simulink model "DetailedModel"  (R2024b)
settings: Solver=ode23t  StartTime=0.0  StopTime=0.2  MaxStep=1e-6  RelTol=1e-4
InitFcn:
  | ModelParameters
undefined symbols (not defined in the file or in its folder): ABR, abr, dc, dc_vs, h_BTU, inv, L, setpoint, Setpoint_Harmonic_L1, time, ts, Ts_RMS
libraries: spsThreePhaseSeriesRLCBranchLib x17, spsGroundLib x14, spsControlledVoltageSourceLib x11, spsThreePhaseVIMeasurementLib x8, spsSeriesRLCBranchLib x7, eePwmGenerator x6, spsCurrentMeasurementLib x4, spsVoltageMeasurementLib x4, spsControlledCurrentSourceLib x3, eePowerMeasurement x3, spsUniversalBridgeLib x2, spsThreePhaseBreakerLib x1
(part 1 of 3)
settings Model: SimulationMode=accelerator  Creator=hw  LastModifiedBy=santh
settings SolverCC: MaxConsecutiveMinStep=10  ShapePreserveControl=EnableAll
settings OptimizationCC: ReuseModelBlockBuffer=off
settings DebuggingCC: UnconnectedInputMsg=warning  UnconnectedOutputMsg=warning  UnconnectedLineMsg=warning
settings ModelReferenceCC: EnableRefExpFcnMdlSchedulingChecks=on
settings RTWCC: GPUComputeCapability=3.5  DLArmComputeVersion=19.05

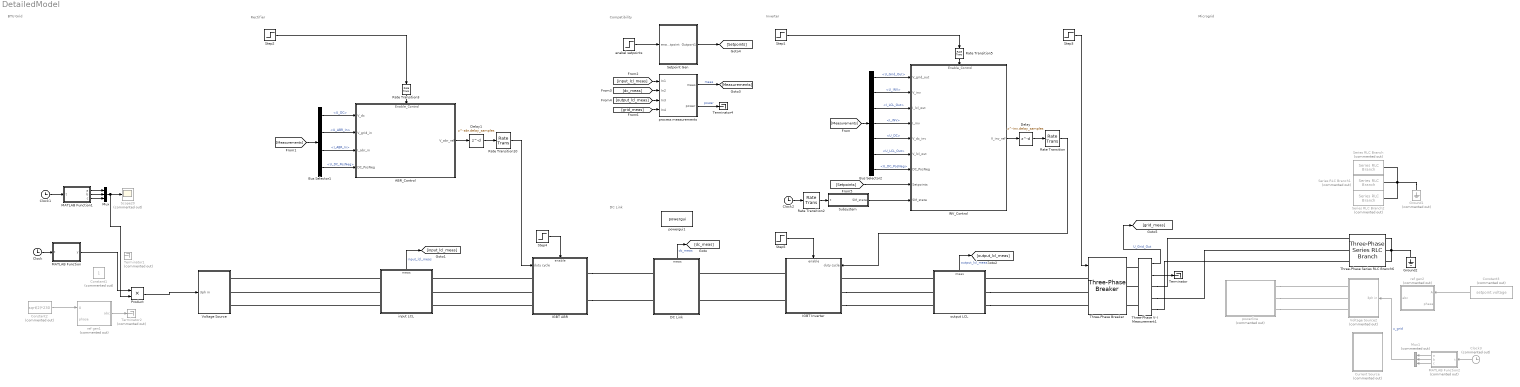
== system DetailedModel ==
  note: Inverter
  note: Rectifier
  note: DC Link
  note: Microgrid
  note: BTU Grid
  note: Compatibility
  " powerline" : Subsystem  Commented=on  Variant=on  VariantControl=Choice
  ABR_Control : Subsystem  Variant=on
      settings: PortSchema="{\"entries\":[{\"content\":{\"sides\":[{\"content\":{\"connectorIds\":[\"In1\",\"In2\",\"In3\",\"In4\"]},\"type\":\"ConnectorPlacement.EquallySpacedRectSide\",\"uuid\":\"9a61e9a7-e233-4fff-bbb7-09c50b9bf7c3\"},{\"content\":{\"connectorIds\":[\"Out1\"],\"side\":\"RIGHT\"},\"type\":\"ConnectorPlacement.EquallySpacedRectSide\",\"uuid\":\"8c6878d7-682c-4532-9753-a6ad9d7eb284\"},{\"content\":{\"connectorIds\":[\"In5\"],\"side\":\"TOP\"},\"type\":\"ConnectorPlacement.EquallySpacedRectSide\",\"uuid\":\"7bdbe081-6677-4104-aee9-21ab386df38d\"}]},\"type\":\"ConnectorPlacement.EquallySpacedConnector\",\"uuid\":\"4e4d951e-f80f-4270-9482-a2bd8c4de465\"}],\"packageUris\":[\"http://schema.mathworks.com/mf0/Connector/R2020b\"],\"version\":\"1.0\"}"
  Bus Selector1 : BusSelector  OutputSignals=U_DC,U_ABR_In,I_ABR_In,U_DC_PosNeg
  Bus Selector2 : BusSelector  OutputSignals=U_Grid_Out,U_INV,I_LCL_Out,I_INV,U_DC,U_LCL_Out,U_DC_PosNeg
  Clock : Clock
  Clock1 : Clock
  Clock2 : Clock
  Clock3 : Clock  Commented=on
  Constant1 : Constant  Commented=on
  Constant2 : Constant  Commented=on  Value=sqrt(2)*230
  Constant3 : Constant  Commented=on  Value=setpoint.voltage
  Current Source : Subsystem  Commented=on  VariantControl=simulate_abr == true;
  DC Link : Subsystem  Variant=on  VariantControl=Choice
      settings: PortSchema="{\"entries\":[{\"content\":{\"sides\":[{\"content\":{\"connectorIds\":[\"LConn1\",\"LConn2\"]},\"type\":\"ConnectorPlacement.EquallySpacedRectSide\",\"uuid\":\"f6ba536e-5264-4926-8f4c-6c75b8afc572\"},{\"content\":{\"connectorIds\":[\"RConn1\",\"RConn2\"],\"side\":\"RIGHT\"},\"type\":\"ConnectorPlacement.EquallySpacedRectSide\",\"uuid\":\"a945ca90-e57b-4883-aff8-0ec279b8e021\"},{\"content\":{\"connectorIds\":[\"Out1\"],\"side\":\"TOP\"},\"type\":\"ConnectorPlacement.EquallySpacedRectSide\",\"uuid\":\"231489ed-e064-4a11-8690-f7178652e5df\"}]},\"type\":\"ConnectorPlacement.EquallySpacedConnector\",\"uuid\":\"69bf4267-a91a-48de-830b-5c3504f7f15c\"}],\"packageUris\":[\"http://schema.mathworks.com/mf0/Connector/R2020b\"],\"version\":\"1.0\"}"
  Delay : Delay  DelayLength=inv.delay_samples
  Delay1 : Delay  DelayLength=abr.delay_samples  SampleTime=h_BTU
  Ground1 : spsGroundLib/Ground  Commented=on  LConnTagsString=a
  Ground2 : spsGroundLib/Ground  LConnTagsString=a
  IGBT ABR : Subsystem  Variant=on  VariantControl=Choice
      settings: PortSchema="{\"entries\":[{\"content\":{\"sides\":[{\"content\":{\"connectorIds\":[\"In1\",\"LConn1\",\"LConn2\",\"LConn3\"]},\"type\":\"ConnectorPlacement.EquallySpacedRectSide\",\"uuid\":\"bdcb7c3b-245c-484b-966a-d1c0a18a3503\"},{\"content\":{\"connectorIds\":[\"RConn1\",\"RConn2\"],\"side\":\"RIGHT\"},\"type\":\"ConnectorPlacement.EquallySpacedRectSide\",\"uuid\":\"68367abd-d947-47d9-a9fd-57ab46e42857\"},{\"content\":{\"connectorIds\":[\"In2\"],\"side\":\"TOP\"},\"type\":\"ConnectorPlacement.EquallySpacedRectSide\",\"uuid\":\"ac48e4a4-8372-427d-a930-cd7797fb7ffc\"}]},\"type\":\"ConnectorPlacement.EquallySpacedConnector\",\"uuid\":\"996b3671-85aa-4bcb-92b7-447b7580701f\"}],\"packageUris\":[\"http://schema.mathworks.com/mf0/Connector/R2020b\"],\"version\":\"1.0\"}"
  IGBT Inverter : Subsystem  Variant=on  VariantControl=Choice
      settings: PortSchema="{\"entries\":[{\"content\":{\"sides\":[{\"content\":{\"connectorIds\":[\"LConn1\",\"LConn2\"]},\"type\":\"ConnectorPlacement.EquallySpacedRectSide\",\"uuid\":\"bdcb7c3b-245c-484b-966a-d1c0a18a3503\"},{\"content\":{\"connectorIds\":[\"In2\",\"RConn1\",\"RConn2\",\"RConn3\"],\"side\":\"RIGHT\"},\"type\":\"ConnectorPlacement.EquallySpacedRectSide\",\"uuid\":\"68367abd-d947-47d9-a9fd-57ab46e42857\"},{\"content\":{\"connectorIds\":[\"In1\"],\"side\":\"TOP\"},\"type\":\"ConnectorPlacement.EquallySpacedRectSide\",\"uuid\":\"ac48e4a4-8372-427d-a930-cd7797fb7ffc\"}]},\"type\":\"ConnectorPlacement.EquallySpacedConnector\",\"uuid\":\"996b3671-85aa-4bcb-92b7-447b7580701f\"}],\"packageUris\":[\"http://schema.mathworks.com/mf0/Connector/R2020b\"],\"version\":\"1.0\"}"
  INV_Control : Subsystem  Variant=on
      settings: PortSchema="{\"entries\":[{\"content\":{\"sides\":[{\"content\":{\"connectorIds\":[\"In1\",\"In2\",\"In3\",\"In4\",\"In5\",\"In6\",\"In7\",\"In8\",\"In9\"]},\"type\":\"ConnectorPlacement.EquallySpacedRectSide\",\"uuid\":\"23e1e123-a779-4f69-b19b-2523a1761b0a\"},{\"content\":{\"connectorIds\":[\"Out1\"],\"side\":\"RIGHT\"},\"type\":\"ConnectorPlacement.EquallySpacedRectSide\",\"uuid\":\"bea06d0c-6610-4352-b580-d1a9b208a554\"},{\"content\":{\"connectorIds\":[\"In10\"],\"side\":\"TOP\"},\"type\":\"ConnectorPlacement.EquallySpacedRectSide\",\"uuid\":\"8bb6373a-e28d-4132-b828-762de06cd811\"}]},\"type\":\"ConnectorPlacement.EquallySpacedConnector\",\"uuid\":\"f1eae18b-7dfa-472c-b275-c02a5c1bef51\"}],\"packageUris\":[\"http://schema.mathworks.com/mf0/Connector/R2020b\"],\"version\":\"1.0\"}"
  MATLAB Function : MATLAB Function  TreatAsAtomicUnit=on
  MATLAB Function1 : MATLAB Function  TreatAsAtomicUnit=on
  MATLAB Function2 : MATLAB Function  Commented=on  TreatAsAtomicUnit=on
  Mux : Mux  Inputs=3
  Mux1 : Mux  Commented=on  Inputs=3
  Product : Product
  Rate Transition : RateTransition
  Rate Transition10 : RateTransition
  Rate Transition2 : RateTransition
  Rate Transition3 : RateTransition  OutPortSampleTime=h_BTU
  Rate Transition5 : RateTransition  OutPortSampleTime=h_BTU
  Scope20 : Scope  Commented=on
  Series RLC Branch : spsSeriesRLCBranchLib/Series RLC Branch  Commented=on  LConnTagsString=__new0  RConnTagsString=__new0  BranchType=R  Resistance=50  Inductance=1e-3  SetiL0=off  InitialCurrent=0  Capacitance=1e-6  Setx0=off  InitialVoltage=0  Measurements=None
  Series RLC Branch1 : spsSeriesRLCBranchLib/Series RLC Branch  Commented=on  LConnTagsString=__new0  RConnTagsString=__new0  BranchType=R  Resistance=40  Inductance=1e-3  SetiL0=off  InitialCurrent=0  Capacitance=1e-6  Setx0=off  InitialVoltage=0  Measurements=None
  Series RLC Branch2 : spsSeriesRLCBranchLib/Series RLC Branch  Commented=on  LConnTagsString=__new0  RConnTagsString=__new0  BranchType=R  Resistance=50  Inductance=1e-3  SetiL0=off  InitialCurrent=0  Capacitance=1e-6  Setx0=off  InitialVoltage=0  Measurements=None
  Setpoint Gen : Subsystem
  Step1 : Step  Time=time.enable_inv_ctrl  SampleTime=0
  Step2 : Step  Time=time.enable_abr_ctrl  SampleTime=0
  Step3 : Step  Time=time.ongrid  SampleTime=0
  Step4 : Step  Time=time.enable_abr  SampleTime=0
  Step5 : Step  Time=time.enable_inv  SampleTime=0
  Subsystem : Subsystem
  Terminator : Terminator
  Terminator1 : Terminator  Commented=on
  Terminator2 : Terminator  Commented=on
  Terminator4 : Terminator
  Three-Phase Series RLC Branch6 : spsThreePhaseSeriesRLCBranchLib/Three-Phase Series RLC Branch  LConnTagsString=A|B|C  RConnTagsString=A|B|C  BranchType=R  Resistance=30  Inductance=350e-6  Capacitance=1e-6  Measurements=None
  Three-Phase V-I Measurement1 : spsThreePhaseVIMeasurementLib/Three-Phase V-I Measurement  VoltageMeasurement=phase-to-ground  SetLabelV=off  LabelV=Vabc  Vpu=off  VpuLL=off  CurrentMeasurement=yes  SetLabelI=off  LabelI=Iabc  Ipu=off  Pbase=100e6  Vbase=500e3  OutputType=Complex  PhasorSimulation=off  PSBequivalent=0
  Three-Phase Breaker : spsThreePhaseBreakerLib/Three-Phase Breaker  InitialState=open  SwitchA=on  SwitchB=on  SwitchC=on  SwitchTimes="[1/60  5/60]"  External=on  BreakerResistance=0.1  SnubberResistance=1e6  SnubberCapacitance=inf  Measurements=None
  Voltage Source : Subsystem  Variant=on  VariantControl=Choice
  Voltage Source2 : Subsystem  Commented=on  VariantControl=simulate_abr == true;
      settings: PortSchema="{\"entries\":[{\"content\":{\"sides\":[{\"content\":{\"connectorIds\":[\"LConn1\",\"LConn2\",\"LConn3\"]},\"type\":\"ConnectorPlacement.EquallySpacedRectSide\",\"uuid\":\"03f06ac6-5cda-41d3-8d94-d4be306d6c6c\"},{\"content\":{\"connectorIds\":[\"In1\"],\"side\":\"RIGHT\"},\"type\":\"ConnectorPlacement.EquallySpacedRectSide\",\"uuid\":\"25d0cb82-e7bd-47db-a03d-611ee4e9a2ac\"},{\"content\":{\"connectorIds\":[],\"side\":\"TOP\"},\"type\":\"ConnectorPlacement.EquallySpacedRectSide\",\"uuid\":\"5bc056cf-5a04-4b34-9ba8-c295df1bce71\"}]},\"type\":\"ConnectorPlacement.EquallySpacedConnector\",\"uuid\":\"225a5fad-493a-40a0-8bfd-b7e904e8dae9\"}],\"packageUris\":[\"http://schema.mathworks.com/mf0/Connector/R2020b\"],\"version\":\"1.0\"}"
  enabel setpoints : Step  Time=time.enable_inv_ctrl  SampleTime=0
  input LCL : Subsystem  Variant=on  VariantControl=Choice
      settings: PortSchema="{\"entries\":[{\"content\":{\"sides\":[{\"content\":{\"connectorIds\":[\"LConn1\",\"LConn2\",\"LConn3\"]},\"type\":\"ConnectorPlacement.EquallySpacedRectSide\",\"uuid\":\"821f425e-e552-4ea9-bdc4-096374f22f7c\"},{\"content\":{\"connectorIds\":[\"RConn1\",\"RConn2\",\"RConn3\"],\"side\":\"RIGHT\"},\"type\":\"ConnectorPlacement.EquallySpacedRectSide\",\"uuid\":\"3ae0e517-8127-4f74-840a-b336b04d9f2b\"},{\"content\":{\"connectorIds\":[\"Out1\"],\"side\":\"TOP\"},\"type\":\"ConnectorPlacement.EquallySpacedRectSide\",\"uuid\":\"969cfcf3-2598-4c06-9b10-5553ede7d6aa\"}]},\"type\":\"ConnectorPlacement.EquallySpacedConnector\",\"uuid\":\"6968de17-154b-4bef-80de-0c55e4fc5823\"}],\"packageUris\":[\"http://schema.mathworks.com/mf0/Connector/R2020b\"],\"version\":\"1.0\"}"
  output LCL : Subsystem
      settings: PortSchema="{\"entries\":[{\"content\":{\"sides\":[{\"content\":{\"connectorIds\":[\"LConn1\",\"LConn2\",\"LConn3\"]},\"type\":\"ConnectorPlacement.EquallySpacedRectSide\",\"uuid\":\"821f425e-e552-4ea9-bdc4-096374f22f7c\"},{\"content\":{\"connectorIds\":[\"RConn1\",\"RConn2\",\"RConn3\"],\"side\":\"RIGHT\"},\"type\":\"ConnectorPlacement.EquallySpacedRectSide\",\"uuid\":\"3ae0e517-8127-4f74-840a-b336b04d9f2b\"},{\"content\":{\"connectorIds\":[\"Out1\"],\"side\":\"TOP\"},\"type\":\"ConnectorPlacement.EquallySpacedRectSide\",\"uuid\":\"969cfcf3-2598-4c06-9b10-5553ede7d6aa\"}]},\"type\":\"ConnectorPlacement.EquallySpacedConnector\",\"uuid\":\"6968de17-154b-4bef-80de-0c55e4fc5823\"}],\"packageUris\":[\"http://schema.mathworks.com/mf0/Connector/R2020b\"],\"version\":\"1.0\"}"
  powergui1 : spspowerguiLib/powergui  Priority=1  SimulationMode=Continuous  SampleTime=h_BTU/100  frequency=60  Iterations=50  frequencyindice=0  Pbase=100e6  ErrMax=1e-4  UnitsV=kV  UnitsW=MW  buscounter=0  FunctionMessages=off  echomessages=off  EnableUseOfTLC=off  CurrentSourceSwitches=off  DisableSnubberDevices=off  DisableRonSwitches=off  DisableVfSwitches=off  DisplayEquations=off  AutomaticDiscreteSolvers=off  SolverType=Tustin/Backward Euler (TBE)  Interpol=off  ExternalGateDelay=off  methode=off  Ts=100  x0status=blocks  SPID=on  SwTol=0  HookPort=off  NonlinearTolerance=1e-4  nMaxIteration=100  ContinueOnMaxIteration=off  RestoreLinks=warning  ResistiveCurrentMeasurement=off  Frange=[0:2:500]  Ylog=off  Xlog=on  ShowGrid=off  save=off  variable=ZData  structure=0  ZoomFFT=off  StartTime=0.0  cycles=1  DisplayStyle=1  fundamental=60  FreqAxis=off  MaxFrequency=1000  frequencyindicesteady=1  RmsSteady=1  display=off
  process measurements : Subsystem
  ref gen1 : Subsystem  Commented=on
  ref gen2 : Subsystem  Commented=on
  wires:
  Delay/1 -> Rate Transition/1
  Step1/1 -> Rate Transition5/1
  Clock1/1 -> MATLAB Function1/1(t)
  Delay1/1 -> Rate Transition10/1
  MATLAB Function1/3(c) -> Mux/3
  Mux/1 -> Product/2, Scope20/1
  ABR_Control/1(V_abr_ref) -> Delay1/1
  MATLAB Function1/2(b) -> Mux/2
  Constant2/1 -> ref gen1/1(A)
  MATLAB Function1/1(a) -> Mux/1
  Clock/1 -> MATLAB Function/1(t)
  INV_Control/1(V_inv_ref) -> Delay/1
  Step2/1 -> Rate Transition3/1
  Rate Transition5/1 -> INV_Control/10(Enable_Control)
  Rate Transition3/1 -> ABR_Control/5(Enable_Control)
  output LCL/1(meas) -> [output_lcl_meas]  "output_lcl_meas"
  [input_lcl_meas] -> process measurements/1(In1)
  [dc_meas] -> process measurements/2(In2)
  [output_lcl_meas] -> process measurements/3(In3)
  DC Link/1(meas) -> [dc_meas]  "dc_meas"
  Bus Selector2/7 -> INV_Control/7(DC_PosNeg)  "<U_DC_PosNeg>"
  Bus Selector2/1 -> INV_Control/1(V_grid_out)  "<U_Grid_Out>"
  Subsystem/1(SM_state) -> INV_Control/9(SM_state)
  Bus Selector1/1 -> ABR_Control/1(V_dc)  "<U_DC>"
  Bus Selector2/3 -> INV_Control/3(I_lcl_out)  "<I_LCL_Out>"
  Bus Selector2/5 -> INV_Control/5(V_dc_inv)  "<U_DC>"
  Bus Selector1/3 -> ABR_Control/3(I_abr_in)  "<I_ABR_In>"
  Bus Selector2/2 -> INV_Control/2(V_inv)  "<U_INV>"
  Bus Selector1/4 -> ABR_Control/4(DC_PosNeg)  "<U_DC_PosNeg>"
  Bus Selector2/4 -> INV_Control/4(I_inv)  "<I_INV>"
  Bus Selector2/6 -> INV_Control/6(V_lcl_out)  "<U_LCL_Out>"
  [Measurements] -> Bus Selector2/1
  Bus Selector1/2 -> ABR_Control/2(V_grid_in)  "<U_ABR_In>"
  process measurements/1(meas) -> [Measurements]  "meas"
  [Setpoints] -> INV_Control/8(Setpoints)
  [Measurements] -> Bus Selector1/1
  Step3/1 -> Three-Phase Breaker/1
  Setpoint Gen/1(Outport1) -> [Setpoints]
  Three-Phase V-I Measurement1/1 -> [grid_meas]  "U_Grid_Out"
  Three-Phase V-I Measurement1/2 -> Terminator/1
  [grid_meas] -> process measurements/4(In4)
  MATLAB Function/1(y) -> Product/1
  ref gen1/1(abc) -> Terminator2/1
  enabel setpoints/1 -> Setpoint Gen/1(enable_setpoint)
  input LCL/1(meas) -> [input_lcl_meas]  "input_lcl_meas"
  Rate Transition10/1 -> IGBT ABR/1(duty cycle)
  Step4/1 -> IGBT ABR/2(enable)
  Rate Transition2/1 -> Subsystem/1(t)
  Clock2/1 -> Rate Transition2/1
  Constant3/1 -> ref gen2/1(A)
  Mux1/1 -> Voltage Source2/1(3ph in)  "u_grid"
  process measurements/2(power) -> Terminator4/1  "power"
  Step5/1 -> IGBT Inverter/1(enable)
  Rate Transition/1 -> IGBT Inverter/2(duty cycle)
  MATLAB Function2/3(c) -> Mux1/3
  MATLAB Function2/2(b) -> Mux1/2
  MATLAB Function2/1(a) -> Mux1/1
  Clock3/1 -> MATLAB Function2/1(t)
  Product/1 -> Voltage Source/1(3ph in)
  connections:
  Three-Phase Series RLC Branch6/RConn1 -- Ground2/LConn1 -- Three-Phase Series RLC Branch6/RConn2 -- Three-Phase Series RLC Branch6/RConn3
  input LCL/LConn1 -- Voltage Source/RConn1
  input LCL/LConn2 -- Voltage Source/RConn2
  input LCL/LConn3 -- Voltage Source/RConn3
  IGBT ABR/LConn1 -- input LCL/RConn1
  IGBT ABR/LConn2 -- input LCL/RConn2
  IGBT ABR/LConn3 -- input LCL/RConn3
  IGBT ABR/RConn1 -- DC Link/LConn1
  IGBT ABR/RConn2 -- DC Link/LConn2
  Three-Phase V-I Measurement1/LConn1 -- Three-Phase Breaker/RConn1
  Three-Phase V-I Measurement1/LConn2 -- Three-Phase Breaker/RConn2
  Three-Phase V-I Measurement1/LConn3 -- Three-Phase Breaker/RConn3
  Three-Phase V-I Measurement1/RConn1 -- Three-Phase Series RLC Branch6/LConn1
  Three-Phase V-I Measurement1/RConn2 -- Three-Phase Series RLC Branch6/LConn2
  Three-Phase V-I Measurement1/RConn3 -- Three-Phase Series RLC Branch6/LConn3
  " powerline"/RConn1 -- Voltage Source2/LConn1
  " powerline"/RConn2 -- Voltage Source2/LConn2
  IGBT Inverter/LConn1 -- DC Link/RConn1
  IGBT Inverter/LConn2 -- DC Link/RConn2
  " powerline"/RConn3 -- Voltage Source2/LConn3
  Ground1/LConn1 -- Series RLC Branch/RConn1 -- Series RLC Branch1/RConn1 -- Series RLC Branch2/RConn1
  output LCL/LConn1 -- IGBT Inverter/RConn1
  IGBT Inverter/RConn2 -- output LCL/LConn2
  IGBT Inverter/RConn3 -- output LCL/LConn3
  Three-Phase Breaker/LConn1 -- output LCL/RConn1
  output LCL/RConn2 -- Three-Phase Breaker/LConn2
  output LCL/RConn3 -- Three-Phase Breaker/LConn3

== system DetailedModel/ powerline ==
  " 0 km" : Subsystem  VariantControl=pimodel == 0
  " 0.5 km" : Subsystem  VariantControl=pimodel == 0.5  mask{L=16e-6, R=20e-3, C=0.56e-6}
      mask prompts: L "Inductance (L)"; R "Resistance (R)"; C "Shunt Capacitys (C)"
  " 10 km" : Subsystem  VariantControl=pimodel == 10  mask{L=350e-6, R=354e-3, C=12e-6}
      mask prompts: L "Inductance (L)"; R "Resistance (R)"; C "Shunt Capacitys (C)"
  " 15 km" : Subsystem  VariantControl=pimodel == 15  mask{L=550e-6, R=538e-3, C=18e-6}
      mask prompts: L "Inductance (L)"; R "Resistance (R)"; C "Shunt Capacitys (C)"
  A1 : PMIOPort  Side=Left
  B1 : PMIOPort  Port=2  Side=Left
  C1 : PMIOPort  Port=3  Side=Left
  A2 : PMIOPort  Port=4  Side=Right
  B2 : PMIOPort  Port=5  Side=Right
  C2 : PMIOPort  Port=6  Side=Right

== system DetailedModel/ABR_Control ==
  note: 1) Add Subsystem or Model blocks as valid variant choices.
      | 2) You cannot connect blocks at this level. At simulation, connectivity is automatically
      | determined, based on the active variant and port name matching.
  V_dc : Inport
  V_grid_in : Inport  Port=2
  I_abr_in : Inport  Port=3
  DC_PosNeg : Inport  Port=4
  Enable_Control : Inport  Port=5
  PR_no_feedback : Subsystem  VariantControl=simulate_abr==true && ABR_Mode == 3  ReferencedSubsystem=PR_no_feedback
  deactive : Subsystem  VariantControl=simulate_abr == false
  V_abr_ref : Outport

== system DetailedModel/Current Source ==
  Constant3 : Constant  Value=setpoint.voltage
  Controlled Current Source1 : spsControlledCurrentSourceLib/Controlled Current Source  Initialize=on  Source_Type=AC  Amplitude=0  Phase=0  Frequency=0  Measurements=None
  Controlled Current Source2 : spsControlledCurrentSourceLib/Controlled Current Source  Initialize=on  Source_Type=AC  Amplitude=0  Phase=0  Frequency=0  Measurements=None
  Controlled Current Source3 : spsControlledCurrentSourceLib/Controlled Current Source  Initialize=on  Source_Type=AC  Amplitude=0  Phase=0  Frequency=0  Measurements=None
  Demux : Demux  Outputs=3
  Divide : Product  Inputs=*/
  Gain : Gain  Gain=setpoint.current
  Ground : spsGroundLib/Ground  LConnTagsString=a
  Terminator : Terminator
  Three-Phase V-I Measurement : spsThreePhaseVIMeasurementLib/Three-Phase V-I Measurement  VoltageMeasurement=phase-to-ground  SetLabelV=off  LabelV=Vabc  Vpu=off  VpuLL=off  CurrentMeasurement=yes  SetLabelI=off  LabelI=Iabc  Ipu=off  Pbase=100e6  Vbase=500e3  OutputType=Complex  PhasorSimulation=off  PSBequivalent=0
  a : PMIOPort  Side=Left
  b : PMIOPort  Port=2  Side=Left
  c : PMIOPort  Port=3  Side=Left
  wires:
  Gain/1 -> Demux/1
  Demux/3 -> Controlled Current Source3/1
  Demux/2 -> Controlled Current Source2/1
  Demux/1 -> Controlled Current Source1/1
  Three-Phase V-I Measurement/2 -> Terminator/1
  Three-Phase V-I Measurement/1 -> Divide/1
  Constant3/1 -> Divide/2
  Divide/1 -> Gain/1
  connections:
  Ground/LConn1 -- Controlled Current Source1/LConn1 -- Controlled Current Source2/LConn1 -- Controlled Current Source3/LConn1
  Controlled Current Source3/RConn1 -- Three-Phase V-I Measurement/LConn3
  Controlled Current Source2/RConn1 -- Three-Phase V-I Measurement/LConn2
  Controlled Current Source1/RConn1 -- Three-Phase V-I Measurement/LConn1
  a/RConn1 -- Three-Phase V-I Measurement/RConn1
  b/RConn1 -- Three-Phase V-I Measurement/RConn2
  c/RConn1 -- Three-Phase V-I Measurement/RConn3

== system DetailedModel/DC Link ==
  full model : Subsystem  VariantControl=simulate_abr == true;
      settings: PortSchema="{\"entries\":[{\"content\":{\"sides\":[{\"content\":{\"connectorIds\":[\"LConn1\",\"LConn2\"]},\"type\":\"ConnectorPlacement.EquallySpacedRectSide\",\"uuid\":\"f6ba536e-5264-4926-8f4c-6c75b8afc572\"},{\"content\":{\"connectorIds\":[\"RConn1\",\"RConn2\"],\"side\":\"RIGHT\"},\"type\":\"ConnectorPlacement.EquallySpacedRectSide\",\"uuid\":\"a945ca90-e57b-4883-aff8-0ec279b8e021\"},{\"content\":{\"connectorIds\":[\"Out1\"],\"side\":\"TOP\"},\"type\":\"ConnectorPlacement.EquallySpacedRectSide\",\"uuid\":\"231489ed-e064-4a11-8690-f7178652e5df\"}]},\"type\":\"ConnectorPlacement.EquallySpacedConnector\",\"uuid\":\"69bf4267-a91a-48de-830b-5c3504f7f15c\"}],\"packageUris\":[\"http://schema.mathworks.com/mf0/Connector/R2020b\"],\"version\":\"1.0\"}"
  vsource : Subsystem  VariantControl=simulate_abr == false;
      settings: PortSchema="{\"entries\":[{\"content\":{\"sides\":[{\"content\":{\"connectorIds\":[\"LConn1\",\"LConn2\"]},\"type\":\"ConnectorPlacement.EquallySpacedRectSide\",\"uuid\":\"f6ba536e-5264-4926-8f4c-6c75b8afc572\"},{\"content\":{\"connectorIds\":[\"RConn1\",\"RConn2\"],\"side\":\"RIGHT\"},\"type\":\"ConnectorPlacement.EquallySpacedRectSide\",\"uuid\":\"a945ca90-e57b-4883-aff8-0ec279b8e021\"},{\"content\":{\"connectorIds\":[\"Out1\"],\"side\":\"TOP\"},\"type\":\"ConnectorPlacement.EquallySpacedRectSide\",\"uuid\":\"231489ed-e064-4a11-8690-f7178652e5df\"}]},\"type\":\"ConnectorPlacement.EquallySpacedConnector\",\"uuid\":\"69bf4267-a91a-48de-830b-5c3504f7f15c\"}],\"packageUris\":[\"http://schema.mathworks.com/mf0/Connector/R2020b\"],\"version\":\"1.0\"}"
  plus1 : PMIOPort  Side=Left
  minus1 : PMIOPort  Port=2  Side=Left
  plus2 : PMIOPort  Port=3  Side=Right
  minus2 : PMIOPort  Port=4  Side=Right
  meas : Outport

== system DetailedModel/IGBT ABR ==
  duty cycle : Inport
  enable : Inport  Port=2
  IGBT ABR : Subsystem  VariantControl=simulate_abr == true;
      settings: PortSchema="{\"entries\":[{\"content\":{\"sides\":[{\"content\":{\"connectorIds\":[\"In1\",\"LConn1\",\"LConn2\",\"LConn3\"]},\"type\":\"ConnectorPlacement.EquallySpacedRectSide\",\"uuid\":\"bdcb7c3b-245c-484b-966a-d1c0a18a3503\"},{\"content\":{\"connectorIds\":[\"RConn1\",\"RConn2\"],\"side\":\"RIGHT\"},\"type\":\"ConnectorPlacement.EquallySpacedRectSide\",\"uuid\":\"68367abd-d947-47d9-a9fd-57ab46e42857\"},{\"content\":{\"connectorIds\":[\"In2\"],\"side\":\"TOP\"},\"type\":\"ConnectorPlacement.EquallySpacedRectSide\",\"uuid\":\"ac48e4a4-8372-427d-a930-cd7797fb7ffc\"}]},\"type\":\"ConnectorPlacement.EquallySpacedConnector\",\"uuid\":\"996b3671-85aa-4bcb-92b7-447b7580701f\"}],\"packageUris\":[\"http://schema.mathworks.com/mf0/Connector/R2020b\"],\"version\":\"1.0\"}"
  deactivate : Subsystem  VariantControl=simulate_abr == false;
      settings: PortSchema="{\"entries\":[{\"content\":{\"sides\":[{\"content\":{\"connectorIds\":[\"In1\",\"LConn1\",\"LConn2\",\"LConn3\"]},\"type\":\"ConnectorPlacement.EquallySpacedRectSide\",\"uuid\":\"bdcb7c3b-245c-484b-966a-d1c0a18a3503\"},{\"content\":{\"connectorIds\":[\"RConn1\",\"RConn2\"],\"side\":\"RIGHT\"},\"type\":\"ConnectorPlacement.EquallySpacedRectSide\",\"uuid\":\"68367abd-d947-47d9-a9fd-57ab46e42857\"},{\"content\":{\"connectorIds\":[\"In2\"],\"side\":\"TOP\"},\"type\":\"ConnectorPlacement.EquallySpacedRectSide\",\"uuid\":\"ac48e4a4-8372-427d-a930-cd7797fb7ffc\"}]},\"type\":\"ConnectorPlacement.EquallySpacedConnector\",\"uuid\":\"996b3671-85aa-4bcb-92b7-447b7580701f\"}],\"packageUris\":[\"http://schema.mathworks.com/mf0/Connector/R2020b\"],\"version\":\"1.0\"}"
  A : PMIOPort  Side=Left
  B : PMIOPort  Port=2  Side=Left
  C : PMIOPort  Port=3  Side=Left
  DC plus : PMIOPort  Port=4  Side=Right
  DC minus : PMIOPort  Port=5  Side=Right

== system DetailedModel/IGBT Inverter ==
  enable : Inport
  duty cycle : Inport  Port=2
  IGBT Inverter : Subsystem  VariantControl="inv_sim_mode == \"igbt\""
      settings: PortSchema="{\"entries\":[{\"content\":{\"sides\":[{\"content\":{\"connectorIds\":[\"LConn1\",\"LConn2\"]},\"type\":\"ConnectorPlacement.EquallySpacedRectSide\",\"uuid\":\"bdcb7c3b-245c-484b-966a-d1c0a18a3503\"},{\"content\":{\"connectorIds\":[\"In2\",\"RConn1\",\"RConn2\",\"RConn3\"],\"side\":\"RIGHT\"},\"type\":\"ConnectorPlacement.EquallySpacedRectSide\",\"uuid\":\"68367abd-d947-47d9-a9fd-57ab46e42857\"},{\"content\":{\"connectorIds\":[\"In1\"],\"side\":\"TOP\"},\"type\":\"ConnectorPlacement.EquallySpacedRectSide\",\"uuid\":\"ac48e4a4-8372-427d-a930-cd7797fb7ffc\"}]},\"type\":\"ConnectorPlacement.EquallySpacedConnector\",\"uuid\":\"996b3671-85aa-4bcb-92b7-447b7580701f\"}],\"packageUris\":[\"http://schema.mathworks.com/mf0/Connector/R2020b\"],\"version\":\"1.0\"}"
  average model : Subsystem  VariantControl="inv_sim_mode == \"avg\""
      settings: PortSchema="{\"entries\":[{\"content\":{\"sides\":[{\"content\":{\"connectorIds\":[\"LConn1\",\"LConn2\"]},\"type\":\"ConnectorPlacement.EquallySpacedRectSide\",\"uuid\":\"bdcb7c3b-245c-484b-966a-d1c0a18a3503\"},{\"content\":{\"connectorIds\":[\"In2\",\"RConn1\",\"RConn2\",\"RConn3\"],\"side\":\"RIGHT\"},\"type\":\"ConnectorPlacement.EquallySpacedRectSide\",\"uuid\":\"68367abd-d947-47d9-a9fd-57ab46e42857\"},{\"content\":{\"connectorIds\":[\"In1\"],\"side\":\"TOP\"},\"type\":\"ConnectorPlacement.EquallySpacedRectSide\",\"uuid\":\"ac48e4a4-8372-427d-a930-cd7797fb7ffc\"}]},\"type\":\"ConnectorPlacement.EquallySpacedConnector\",\"uuid\":\"996b3671-85aa-4bcb-92b7-447b7580701f\"}],\"packageUris\":[\"http://schema.mathworks.com/mf0/Connector/R2020b\"],\"version\":\"1.0\"}"
  DC plus : PMIOPort  Side=Left
  DC minus : PMIOPort  Port=2  Side=Left
  A : PMIOPort  Port=3  Side=Right
  B : PMIOPort  Port=4  Side=Right
  C : PMIOPort  Port=5  Side=Right

== system DetailedModel/INV_Control ==
  note: 1) Add Subsystem or Model blocks as valid variant choices.
      | 2) You cannot connect blocks at this level. At simulation, connectivity is automatically
      | determined, based on the active variant and port name matching.
  V_grid_out : Inport
  V_inv : Inport  Port=2
  I_lcl_out : Inport  Port=3
  I_inv : Inport  Port=4
  V_dc_inv : Inport  Port=5
  V_lcl_out : Inport  Port=6
  DC_PosNeg : Inport  Port=7
  Setpoints : Inport  Port=8
  SM_state : Inport  Port=9
  Enable_Control : Inport  Port=10
  BTU_DQ_Current_Control : Subsystem  VariantControl=INV_Mode==10  ReferencedSubsystem=BTU_DQ_Current_Control
      settings: PortSchema="{\"entries\":[{\"content\":{\"sides\":[{\"content\":{\"connectorIds\":[\"In9\",\"In10\",\"In1\",\"In2\",\"In3\",\"In4\",\"In5\",\"In6\",\"In7\",\"In8\"]},\"type\":\"ConnectorPlacement.EquallySpacedRectSide\",\"uuid\":\"6baa388e-7184-42e1-a65e-c042756fabf1\"},{\"content\":{\"connectorIds\":[\"Out1\"],\"side\":\"RIGHT\"},\"type\":\"ConnectorPlacement.EquallySpacedRectSide\",\"uuid\":\"9ce0a75c-01ec-48aa-a778-a1584ec40358\"},{\"content\":{\"side\":\"TOP\"},\"type\":\"ConnectorPlacement.EquallySpacedRectSide\",\"uuid\":\"441b7bcf-f48e-499e-91f5-94fbdb47275e\"}]},\"type\":\"ConnectorPlacement.EquallySpacedConnector\",\"uuid\":\"4bbbbfed-a9b6-439f-a0bf-aea6944f8f31\"}],\"packageUris\":[\"http://schema.mathworks.com/mf0/Connector/R2020b\"],\"version\":\"1.0\"}"
  BTU_DQ_Voltage_Control : Subsystem  VariantControl=INV_Mode==9  ReferencedSubsystem=BTU_DQ_Voltage_Control
  BTU_Droop_DQ_based : Subsystem  VariantControl=INV_Mode==11  ReferencedSubsystem=BTU_Droop_DQ_based
      settings: PortSchema="{\"entries\":[{\"content\":{\"sides\":[{\"content\":{\"connectorIds\":[\"In9\",\"In10\",\"In1\",\"In2\",\"In3\",\"In4\",\"In5\",\"In6\",\"In7\",\"In8\"]},\"type\":\"ConnectorPlacement.EquallySpacedRectSide\",\"uuid\":\"6baa388e-7184-42e1-a65e-c042756fabf1\"},{\"content\":{\"connectorIds\":[\"Out1\"],\"side\":\"RIGHT\"},\"type\":\"ConnectorPlacement.EquallySpacedRectSide\",\"uuid\":\"9ce0a75c-01ec-48aa-a778-a1584ec40358\"},{\"content\":{\"side\":\"TOP\"},\"type\":\"ConnectorPlacement.EquallySpacedRectSide\",\"uuid\":\"441b7bcf-f48e-499e-91f5-94fbdb47275e\"}]},\"type\":\"ConnectorPlacement.EquallySpacedConnector\",\"uuid\":\"4bbbbfed-a9b6-439f-a0bf-aea6944f8f31\"}],\"packageUris\":[\"http://schema.mathworks.com/mf0/Connector/R2020b\"],\"version\":\"1.0\"}"
  BTU_PR_Current_Control : Subsystem  VariantControl=INV_Mode==8  ReferencedSubsystem=BTU_PR_Current_Control
  BTU_PR_Voltage_Control : Subsystem  VariantControl=INV_Mode==7  ReferencedSubsystem=BTU_PR_Voltage_Control
  V_inv_ref : Outport

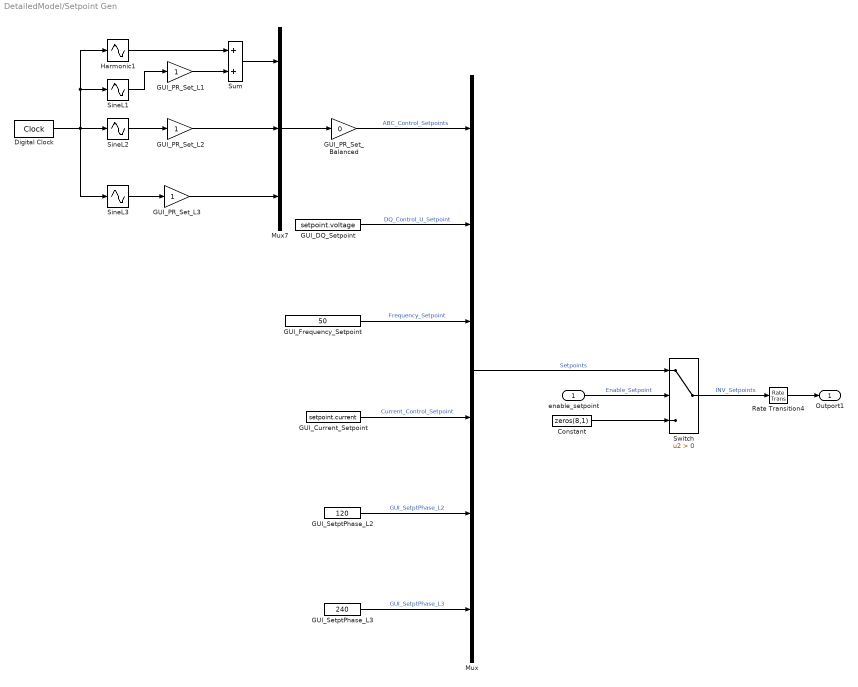
== system DetailedModel/Setpoint Gen ==
  enable_setpoint : Inport
  Constant : Constant  Value=zeros(8,1)  SampleTime=-1
  Digital Clock : DigitalClock  SampleTime=h_BTU
  GUI_Current_Setpoint : Constant  Value=setpoint.current  SampleTime=-1
  GUI_DQ_Setpoint : Constant  Value=setpoint.voltage  SampleTime=-1
  GUI_Frequency_Setpoint : Constant  Value=50  SampleTime=-1
  GUI_PR_Set_Balanced : Gain  Gain=0
  GUI_PR_Set_L1 : Gain
  GUI_PR_Set_L2 : Gain
  GUI_PR_Set_L3 : Gain
  GUI_SetptPhase_L2 : Constant  Value=120  SampleTime=-1
  GUI_SetptPhase_L3 : Constant  Value=240  SampleTime=-1
  Harmonic1 : Sin  TimeSource=Use external signal  Amplitude=Setpoint_Harmonic_L1  Frequency=2*pi*50*7
  Mux : Mux  Inputs=6
  Mux7 : Mux  Inputs=3
  Rate Transition4 : RateTransition  OutPortSampleTime=h_BTU
  SineL1 : Sin  TimeSource=Use external signal  Frequency=2*pi*50
  SineL2 : Sin  TimeSource=Use external signal  Frequency=2*pi*50  Phase=-2*pi/3
  SineL3 : Sin  TimeSource=Use external signal  Frequency=2*pi*50  Phase=-2*pi*2/3
  Sum : Sum
  Switch : Switch  Criteria=u2 > Threshold  SaturateOnIntegerOverflow=off  InputSameDT=off
  Outport1 : Outport
  wires:
  Mux7/1 -> GUI_PR_Set_Balanced/1
  SineL2/1 -> GUI_PR_Set_L2/1
  SineL3/1 -> GUI_PR_Set_L3/1
  SineL1/1 -> GUI_PR_Set_L1/1
  GUI_Current_Setpoint/1 -> Mux/4  "Current_Control_Setpoint"
  GUI_PR_Set_Balanced/1 -> Mux/1  "ABC_Control_Setpoints"
  GUI_PR_Set_L1/1 -> Sum/2
  GUI_PR_Set_L2/1 -> Mux7/2
  GUI_PR_Set_L3/1 -> Mux7/3
  GUI_Frequency_Setpoint/1 -> Mux/3  "Frequency_Setpoint"
  GUI_DQ_Setpoint/1 -> Mux/2  "DQ_Control_U_Setpoint"
  Mux/1 -> Switch/1  "Setpoints"
  Digital Clock/1 -> SineL3/1, Harmonic1/1, SineL1/1, SineL2/1
  Harmonic1/1 -> Sum/1
  Sum/1 -> Mux7/1
  GUI_SetptPhase_L2/1 -> Mux/5  "GUI_SetptPhase_L2"
  GUI_SetptPhase_L3/1 -> Mux/6  "GUI_SetptPhase_L3"
  Constant/1 -> Switch/3
  enable_setpoint/1 -> Switch/2  "Enable_Setpoint"
  Switch/1 -> Rate Transition4/1  "INV_Setpoints"
  Rate Transition4/1 -> Outport1/1

== system DetailedModel/Subsystem ==
  t : Inport
  Constant : Constant  Value=time.ongrid
  Constant1 : Constant  Value=6
  Constant2 : Constant  Value=time.enable_abr
  Constant3 : Constant  Value=5
  Constant4 : Constant  Value=4
  GreaterThanOrEqual : RelationalOperator  OutDataTypeStr=boolean  RndMeth=Simplest  InputSameDT=off
  GreaterThanOrEqual1 : RelationalOperator  OutDataTypeStr=boolean  RndMeth=Simplest  InputSameDT=off
  Switch : Switch  Criteria=u2 > Threshold  SaturateOnIntegerOverflow=off  InputSameDT=off
  Switch1 : Switch  Criteria=u2 > Threshold  SaturateOnIntegerOverflow=off  InputSameDT=off
  SM_state : Outport
  wires:
  Constant/1 -> GreaterThanOrEqual/2
  GreaterThanOrEqual/1 -> Switch/2
  Constant1/1 -> Switch/1
  GreaterThanOrEqual1/1 -> Switch1/2
  Constant3/1 -> Switch1/1
  t/1 -> GreaterThanOrEqual1/1, GreaterThanOrEqual/1
  Constant2/1 -> GreaterThanOrEqual1/2
  Switch1/1 -> Switch/3
  Constant4/1 -> Switch1/3
  Switch/1 -> SM_state/1

== system DetailedModel/Voltage Source ==
  3ph in : Inport
  Voltage Source : Subsystem  VariantControl=simulate_abr == true;
  deactive : Subsystem  VariantControl=simulate_abr == false;
  a : PMIOPort  Side=Right
  b : PMIOPort  Port=2  Side=Right
  c : PMIOPort  Port=3  Side=Right

== system DetailedModel/Voltage Source2 ==
  3ph in : Inport
  Controlled Voltage Source : spsControlledVoltageSourceLib/Controlled Voltage Source  Initialize=on  Source_Type=AC  Amplitude=0  Phase=0  Frequency=0  Measurements=None
  Controlled Voltage Source1 : spsControlledVoltageSourceLib/Controlled Voltage Source  Initialize=on  Source_Type=AC  Amplitude=0  Phase=0  Frequency=0  Measurements=None
  Controlled Voltage Source2 : spsControlledVoltageSourceLib/Controlled Voltage Source  Initialize=on  Source_Type=AC  Amplitude=0  Phase=0  Frequency=0  Measurements=None
  Demux : Demux  Outputs=3
  Ground : spsGroundLib/Ground  LConnTagsString=a
  Three-Phase Series RLC Branch1 : spsThreePhaseSeriesRLCBranchLib/Three-Phase Series RLC Branch  LConnTagsString=A|B|C  RConnTagsString=A|B|C  BranchType=R  Resistance=1e-4  Inductance=L  Capacitance=1e-6  Measurements=None
  a : PMIOPort  Side=Left
  b : PMIOPort  Port=2  Side=Left
  c : PMIOPort  Port=3  Side=Left
  wires:
  3ph in/1 -> Demux/1
  Demux/3 -> Controlled Voltage Source2/1
  Demux/2 -> Controlled Voltage Source1/1
  Demux/1 -> Controlled Voltage Source/1
  connections:
  Three-Phase Series RLC Branch1/LConn3 -- Controlled Voltage Source2/RConn1
  Three-Phase Series RLC Branch1/LConn2 -- Controlled Voltage Source1/RConn1
  Three-Phase Series RLC Branch1/LConn1 -- Controlled Voltage Source/RConn1
  Ground/LConn1 -- Controlled Voltage Source1/LConn1 -- Controlled Voltage Source2/LConn1 -- Controlled Voltage Source/LConn1
  c/RConn1 -- Three-Phase Series RLC Branch1/RConn3
  Three-Phase Series RLC Branch1/RConn2 -- b/RConn1
  Three-Phase Series RLC Branch1/RConn1 -- a/RConn1

== system DetailedModel/input LCL ==
  deactive : Subsystem  VariantControl=simulate_abr == false
      settings: PortSchema="{\"entries\":[{\"content\":{\"sides\":[{\"content\":{\"connectorIds\":[\"LConn1\",\"LConn2\",\"LConn3\"]},\"type\":\"ConnectorPlacement.EquallySpacedRectSide\",\"uuid\":\"821f425e-e552-4ea9-bdc4-096374f22f7c\"},{\"content\":{\"connectorIds\":[\"RConn1\",\"RConn2\",\"RConn3\"],\"side\":\"RIGHT\"},\"type\":\"ConnectorPlacement.EquallySpacedRectSide\",\"uuid\":\"3ae0e517-8127-4f74-840a-b336b04d9f2b\"},{\"content\":{\"connectorIds\":[\"Out1\"],\"side\":\"TOP\"},\"type\":\"ConnectorPlacement.EquallySpacedRectSide\",\"uuid\":\"969cfcf3-2598-4c06-9b10-5553ede7d6aa\"}]},\"type\":\"ConnectorPlacement.EquallySpacedConnector\",\"uuid\":\"6968de17-154b-4bef-80de-0c55e4fc5823\"}],\"packageUris\":[\"http://schema.mathworks.com/mf0/Connector/R2020b\"],\"version\":\"1.0\"}"
  input LCL : Subsystem  VariantControl=simulate_abr == true
      settings: PortSchema="{\"entries\":[{\"content\":{\"sides\":[{\"content\":{\"connectorIds\":[\"LConn1\",\"LConn2\",\"LConn3\"]},\"type\":\"ConnectorPlacement.EquallySpacedRectSide\",\"uuid\":\"821f425e-e552-4ea9-bdc4-096374f22f7c\"},{\"content\":{\"connectorIds\":[\"RConn1\",\"RConn2\",\"RConn3\"],\"side\":\"RIGHT\"},\"type\":\"ConnectorPlacement.EquallySpacedRectSide\",\"uuid\":\"3ae0e517-8127-4f74-840a-b336b04d9f2b\"},{\"content\":{\"connectorIds\":[\"Out1\"],\"side\":\"TOP\"},\"type\":\"ConnectorPlacement.EquallySpacedRectSide\",\"uuid\":\"969cfcf3-2598-4c06-9b10-5553ede7d6aa\"}]},\"type\":\"ConnectorPlacement.EquallySpacedConnector\",\"uuid\":\"6968de17-154b-4bef-80de-0c55e4fc5823\"}],\"packageUris\":[\"http://schema.mathworks.com/mf0/Connector/R2020b\"],\"version\":\"1.0\"}"
  A1 : PMIOPort  Side=Left
  B1 : PMIOPort  Port=2  Side=Left
  C1 : PMIOPort  Port=3  Side=Left
  A2 : PMIOPort  Port=4  Side=Right
  B2 : PMIOPort  Port=5  Side=Right
  C2 : PMIOPort  Port=6  Side=Right
  meas : Outport

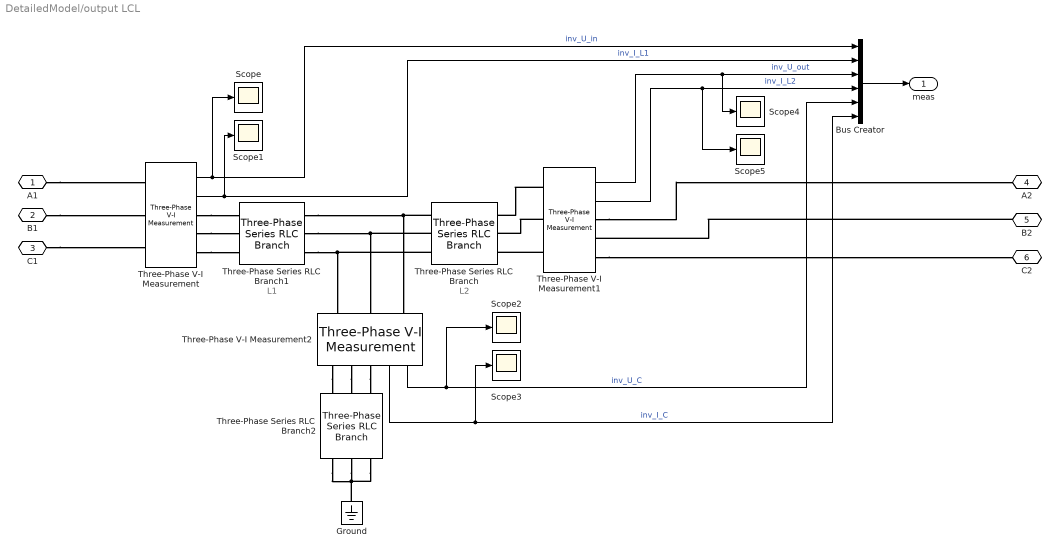
== system DetailedModel/output LCL ==
  note: L2
  note: L1
  Bus Creator : BusCreator  Inputs=6
  Ground : spsGroundLib/Ground  LConnTagsString=a
  Scope{,1..5} (6 alike) : Scope
  Three-Phase Series RLC Branch : spsThreePhaseSeriesRLCBranchLib/Three-Phase Series RLC Branch  LConnTagsString=A|B|C  RConnTagsString=A|B|C  BranchType=RL  Resistance=inv.R2  Inductance=inv.L2  Capacitance=1e-6  Measurements=None
  Three-Phase Series RLC Branch1 : spsThreePhaseSeriesRLCBranchLib/Three-Phase Series RLC Branch  LConnTagsString=A|B|C  RConnTagsString=A|B|C  BranchType=RL  Resistance=inv.R1  Inductance=inv.L1  Capacitance=1e-6  Measurements=None
  Three-Phase Series RLC Branch2 : spsThreePhaseSeriesRLCBranchLib/Three-Phase Series RLC Branch  LConnTagsString=A|B|C  RConnTagsString=A|B|C  BranchType=RC  Resistance=inv.RC  Inductance=13e-6  Capacitance=inv.C  Measurements=None
  Three-Phase V-I Measurement : spsThreePhaseVIMeasurementLib/Three-Phase V-I Measurement  VoltageMeasurement=phase-to-ground  SetLabelV=off  LabelV=Vabc  Vpu=off  VpuLL=off  CurrentMeasurement=yes  SetLabelI=off  LabelI=Iabc  Ipu=off  Pbase=100e6  Vbase=500e3  OutputType=Complex  PhasorSimulation=off  PSBequivalent=0
  Three-Phase V-I Measurement1 : spsThreePhaseVIMeasurementLib/Three-Phase V-I Measurement  VoltageMeasurement=phase-to-ground  SetLabelV=off  LabelV=Vabc  Vpu=off  VpuLL=off  CurrentMeasurement=yes  SetLabelI=off  LabelI=Iabc  Ipu=off  Pbase=100e6  Vbase=500e3  OutputType=Complex  PhasorSimulation=off  PSBequivalent=0
  Three-Phase V-I Measurement2 : spsThreePhaseVIMeasurementLib/Three-Phase V-I Measurement  VoltageMeasurement=phase-to-ground  SetLabelV=off  LabelV=Vabc  Vpu=off  VpuLL=off  CurrentMeasurement=yes  SetLabelI=off  LabelI=Iabc  Ipu=off  Pbase=100e6  Vbase=500e3  OutputType=Complex  PhasorSimulation=off  PSBequivalent=0
  A1 : PMIOPort  Side=Left
  B1 : PMIOPort  Port=2  Side=Left
  C1 : PMIOPort  Port=3  Side=Left
  A2 : PMIOPort  Port=4  Side=Right
  B2 : PMIOPort  Port=5  Side=Right
  C2 : PMIOPort  Port=6  Side=Right
  meas : Outport
  wires:
  Bus Creator/1 -> meas/1
  Three-Phase V-I Measurement1/2 -> Scope5/1, Bus Creator/4  "inv_I_L2"
  Three-Phase V-I Measurement/2 -> Scope1/1, Bus Creator/2  "inv_I_L1"
  Three-Phase V-I Measurement/1 -> Scope/1, Bus Creator/1  "inv_U_in"
  Three-Phase V-I Measurement2/1 -> Scope2/1, Bus Creator/5  "inv_U_C"
  Three-Phase V-I Measurement2/2 -> Scope3/1, Bus Creator/6  "inv_I_C"
  Three-Phase V-I Measurement1/1 -> Scope4/1, Bus Creator/3  "inv_U_out"
  connections:
  Three-Phase V-I Measurement1/RConn3 -- C2/RConn1
  B2/RConn1 -- Three-Phase V-I Measurement1/RConn2
  B1/RConn1 -- Three-Phase V-I Measurement/LConn2
  Three-Phase V-I Measurement2/RConn2 -- Three-Phase Series RLC Branch2/LConn2
  Three-Phase Series RLC Branch/LConn1 -- Three-Phase Series RLC Branch1/RConn1 -- Three-Phase V-I Measurement2/LConn1
  Three-Phase V-I Measurement1/LConn2 -- Three-Phase Series RLC Branch/RConn2
  Three-Phase V-I Measurement2/RConn1 -- Three-Phase Series RLC Branch2/LConn3
  A1/RConn1 -- Three-Phase V-I Measurement/LConn1
  Three-Phase Series RLC Branch/LConn2 -- Three-Phase Series RLC Branch1/RConn2 -- Three-Phase V-I Measurement2/LConn2
  Three-Phase V-I Measurement1/LConn3 -- Three-Phase Series RLC Branch/RConn3
  C1/RConn1 -- Three-Phase V-I Measurement/LConn3
  Three-Phase Series RLC Branch/LConn3 -- Three-Phase Series RLC Branch1/RConn3 -- Three-Phase V-I Measurement2/LConn3
  Three-Phase V-I Measurement1/RConn1 -- A2/RConn1
  Three-Phase V-I Measurement1/LConn1 -- Three-Phase Series RLC Branch/RConn1
  Three-Phase V-I Measurement2/RConn3 -- Three-Phase Series RLC Branch2/LConn1
  Three-Phase Series RLC Branch2/RConn2 -- Three-Phase Series RLC Branch2/RConn1 -- Ground/LConn1 -- Three-Phase Series RLC Branch2/RConn3
  Three-Phase V-I Measurement/RConn3 -- Three-Phase Series RLC Branch1/LConn3
  Three-Phase V-I Measurement/RConn2 -- Three-Phase Series RLC Branch1/LConn2
  Three-Phase V-I Measurement/RConn1 -- Three-Phase Series RLC Branch1/LConn1

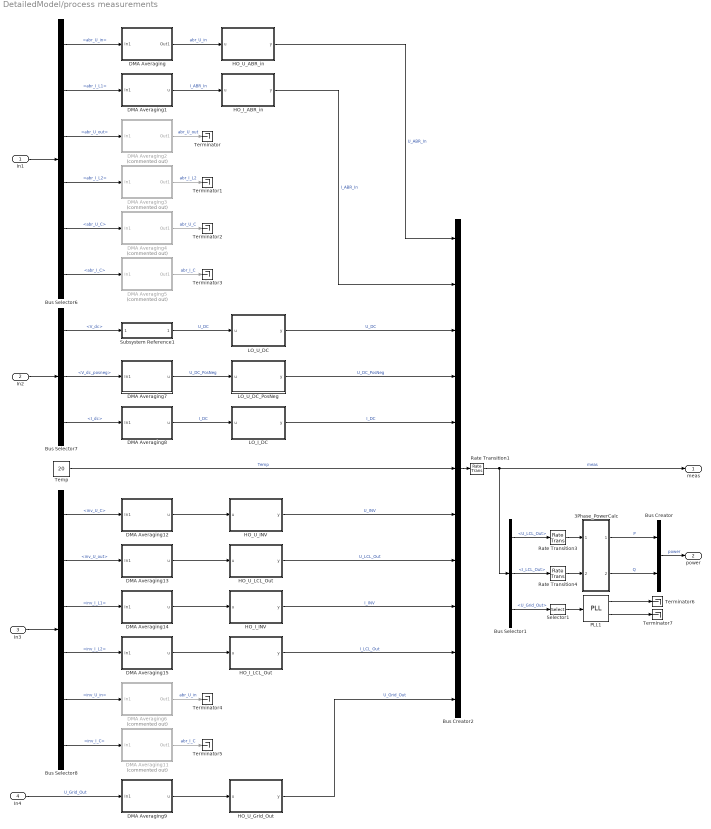
== system DetailedModel/process measurements ==
  In1 : Inport
  In2 : Inport  Port=2
  In3 : Inport  Port=3
  In4 : Inport  Port=4
  3Phase_PowerCalc : Subsystem
  Bus Creator : BusCreator  Inputs=2
  Bus Creator2 : BusCreator  Inputs=11
  Bus Selector1 : BusSelector  OutputSignals=U_LCL_Out,I_LCL_Out,U_Grid_Out
  Bus Selector6 : BusSelector  OutputSignals=abr_U_in,abr_I_L1,abr_U_out,abr_I_L2,abr_U_C,abr_I_C
  Bus Selector7 : BusSelector  OutputSignals=V_dc,V_dc_posneg,I_dc
  Bus Selector8 : BusSelector  OutputSignals=inv_U_C,inv_U_out,inv_I_L1,inv_I_L2,inv_U_in,inv_I_C
  DMA Averaging : Subsystem
  DMA Averaging1 : Subsystem
  DMA Averaging11 : Subsystem  Commented=on
  DMA Averaging12 : Subsystem
  DMA Averaging13 : Subsystem
  DMA Averaging14 : Subsystem
  DMA Averaging15 : Subsystem
  DMA Averaging2 : Subsystem  Commented=on
  DMA Averaging3 : Subsystem  Commented=on
  DMA Averaging4 : Subsystem  Commented=on
  DMA Averaging5 : Subsystem  Commented=on
  DMA Averaging6 : Subsystem  Commented=on
  DMA Averaging7 : Subsystem
  DMA Averaging8 : Subsystem
  DMA Averaging9 : Subsystem
  HO_I_ABR_in : Subsystem  Variant=on  VariantControl=Choice
  HO_I_INV : Subsystem  Variant=on  VariantControl=Choice
  HO_I_LCL_Out : Subsystem  Variant=on  VariantControl=Choice
  HO_U_ABR_in : Subsystem  Variant=on  VariantControl=Choice
  HO_U_Grid_Out : Subsystem  Variant=on  VariantControl=Choice
  HO_U_INV : Subsystem  Variant=on  VariantControl=Choice
  HO_U_LCL_Out : Subsystem  Variant=on  VariantControl=Choice
  LO_I_DC : Subsystem  Variant=on  VariantControl=Choice
  LO_U_DC : Subsystem  Variant=on  VariantControl=Choice
  LO_U_DC_PosNeg : Subsystem  Variant=on  VariantControl=Choice
  PLL1 : spsPLLLib/PLL  Fmin=40  Par_Init=[0, 50]  ParK=[100, 1800, 0.7]  TcD=ts*4  MaxRateChangeFreq=12  FilterCutOffFreq=25  Ts=ts  AGC=on
  Rate Transition1 : RateTransition  OutPortSampleTime=h_BTU
  Rate Transition3 : RateTransition  OutPortSampleTimeMultiple=Ts_RMS  OutPortSampleTime=Ts_RMS
  Rate Transition4 : RateTransition  OutPortSampleTimeMultiple=Ts_RMS  OutPortSampleTime=Ts_RMS
  Selector1 : Selector  InputPortWidth=3  IndexOptions=Index vector (dialog)  Indices=[1]  OutputSizes=1
  Subsystem Reference1 : Subsystem  ReferencedSubsystem=DMA_frame_average  samplerate=h_BTU  framesize=DMA_framesize
  Temp : Constant  Value=20
  Terminator{,1..7} (8 alike) : Terminator
  meas : Outport
  power : Outport  Port=2
  wires:
  In3/1 -> Bus Selector8/1
  In1/1 -> Bus Selector6/1
  LO_I_DC/1(y) -> Bus Creator2/5  "I_DC"
  DMA Averaging8/1(u) -> LO_I_DC/1(u)  "I_DC"
  DMA Averaging1/1(u) -> HO_I_ABR_in/1(u)  "I_ABR_In"
  HO_I_LCL_Out/1(y) -> Bus Creator2/10  "I_LCL_Out"
  DMA Averaging14/1(u) -> HO_I_INV/1(u)
  DMA Averaging12/1(u) -> HO_U_INV/1(u)
  HO_U_LCL_Out/1(y) -> Bus Creator2/8  "U_LCL_Out"
  DMA Averaging13/1(u) -> HO_U_LCL_Out/1(u)
  HO_U_ABR_in/1(y) -> Bus Creator2/1  "U_ABR_In"
  Bus Selector8/3 -> DMA Averaging14/1(In1)  "<inv_I_L1>"
  DMA Averaging15/1(u) -> HO_I_LCL_Out/1(u)
  DMA Averaging3/1(Out1) -> Terminator1/1  "abr_I_L2"
  DMA Averaging/1(Out1) -> HO_U_ABR_in/1(u)  "abr_U_in"
  DMA Averaging11/1(Out1) -> Terminator5/1  "abr_I_C"
  Bus Selector6/2 -> DMA Averaging1/1(In1)  "<abr_I_L1>"
  Bus Selector8/1 -> DMA Averaging12/1(In1)  "<inv_U_C>"
  LO_U_DC_PosNeg/1(y) -> Bus Creator2/4  "U_DC_PosNeg"
  HO_I_ABR_in/1(y) -> Bus Creator2/2  "I_ABR_In"
  In2/1 -> Bus Selector7/1
  LO_U_DC/1(y) -> Bus Creator2/3  "U_DC"
  Bus Selector8/5 -> DMA Averaging6/1(In1)  "<inv_U_in>"
  Subsystem Reference1/1 -> LO_U_DC/1(u)  "U_DC"
  Bus Selector8/6 -> DMA Averaging11/1(In1)  "<inv_I_C>"
  HO_U_INV/1(y) -> Bus Creator2/7  "U_INV"
  HO_I_INV/1(y) -> Bus Creator2/9  "I_INV"
  DMA Averaging4/1(Out1) -> Terminator2/1  "abr_U_C"
  DMA Averaging5/1(Out1) -> Terminator3/1  "abr_I_C"
  Bus Selector6/3 -> DMA Averaging2/1(In1)  "<abr_U_out>"
  Bus Selector7/3 -> DMA Averaging8/1(In1)  "<I_dc>"
  Bus Selector6/5 -> DMA Averaging4/1(In1)  "<abr_U_C>"
  Bus Selector8/2 -> DMA Averaging13/1(In1)  "<inv_U_out>"
  Bus Selector7/2 -> DMA Averaging7/1(In1)  "<V_dc_posneg>"
  DMA Averaging6/1(Out1) -> Terminator4/1  "abr_U_in"
  Bus Selector7/1 -> Subsystem Reference1/1  "<V_dc>"
  Bus Selector6/4 -> DMA Averaging3/1(In1)  "<abr_I_L2>"
  Bus Selector6/1 -> DMA Averaging/1(In1)  "<abr_U_in>"
  DMA Averaging2/1(Out1) -> Terminator/1  "abr_U_out"
  Bus Selector6/6 -> DMA Averaging5/1(In1)  "<abr_I_C>"
  Bus Selector8/4 -> DMA Averaging15/1(In1)  "<inv_I_L2>"
  Temp/1 -> Bus Creator2/6  "Temp"
  DMA Averaging7/1(u) -> LO_U_DC_PosNeg/1(u)  "U_DC_PosNeg"
  In4/1 -> DMA Averaging9/1(In1)  "U_Grid_Out"
  DMA Averaging9/1(u) -> HO_U_Grid_Out/1(u)
  HO_U_Grid_Out/1(y) -> Bus Creator2/11  "U_Grid_Out"
  Rate Transition3/1 -> 3Phase_PowerCalc/1(Inport)
  Bus Selector1/2 -> Rate Transition4/1  "<I_LCL_Out>"
  Bus Selector1/3 -> Selector1/1  "<U_Grid_Out>"
  PLL1/1 -> Terminator6/1
  3Phase_PowerCalc/2(Outport2) -> Bus Creator/2  "Q"
  Selector1/1 -> PLL1/1
  Bus Selector1/1 -> Rate Transition3/1  "<U_LCL_Out>"
  Rate Transition4/1 -> 3Phase_PowerCalc/2(Inport2)
  PLL1/2 -> Terminator7/1
  3Phase_PowerCalc/1(Outport) -> Bus Creator/1  "P"
  Bus Creator/1 -> power/1  "power"
  Bus Creator2/1 -> Rate Transition1/1
  Rate Transition1/1 -> Bus Selector1/1, meas/1  "meas"

== system DetailedModel/ref gen1 ==
  A : Inport
  phase : Inport  Port=2
  Constant : Constant  Value=2/3*pi
  Constant1 : Constant  Value=4/3*pi
  Mux : Mux  Inputs=3
  Product : Product
  Product1 : Product
  Product2 : Product
  Ramp : simulink/Sources/Ramp  slope=2*pi*50  start=0  InitialOutput=0
  Sum : Sum  Inputs=+-|
  Sum1 : Sum  Inputs=+-|
  Sum2 : Sum  Inputs=++|
  Trigonometric Function : Trigonometry  Operator=cos
  Trigonometric Function1 : Trigonometry  Operator=cos
  Trigonometric Function2 : Trigonometry  Operator=cos
  abc : Outport
  wires:
  phase/1 -> Sum2/2
  Ramp/1 -> Sum2/1
  Constant1/1 -> Sum1/2
  Constant/1 -> Sum/2
  Mux/1 -> abc/1
  A/1 -> Product2/1, Product1/1, Product/1
  Product/1 -> Mux/1
  Product1/1 -> Mux/2
  Product2/1 -> Mux/3
  Trigonometric Function2/1 -> Product2/2
  Trigonometric Function1/1 -> Product1/2
  Trigonometric Function/1 -> Product/2
  Sum1/1 -> Trigonometric Function2/1
  Sum/1 -> Trigonometric Function1/1
  Sum2/1 -> Sum/1, Sum1/1, Trigonometric Function/1

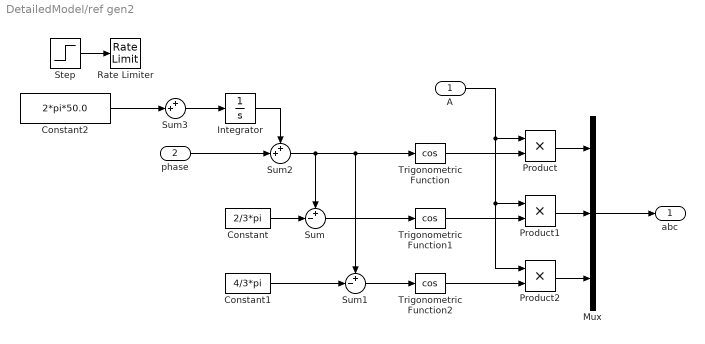
== system DetailedModel/ref gen2 ==
  A : Inport
  phase : Inport  Port=2
  Constant : Constant  Value=2/3*pi
  Constant1 : Constant  Value=4/3*pi
  Constant2 : Constant  Value=2*pi*50.0
  Integrator : Integrator
  Mux : Mux  Inputs=3
  Product : Product
  Product1 : Product
  Product2 : Product
  Rate Limiter : RateLimiter  RisingSlewLimit=0.01  FallingSlewLimit=-0.01  SampleTimeMode=inherited
  Step : Step  Time=2  After=0.01  SampleTime=0
  Sum : Sum  Inputs=+-|
  Sum1 : Sum  Inputs=+-|
  Sum2 : Sum  Inputs=++|
  Sum3 : Sum  Inputs=++|
  Trigonometric Function : Trigonometry  Operator=cos
  Trigonometric Function1 : Trigonometry  Operator=cos
  Trigonometric Function2 : Trigonometry  Operator=cos
  abc : Outport
  wires:
  phase/1 -> Sum2/2
  Constant1/1 -> Sum1/2
  Constant/1 -> Sum/2
  Mux/1 -> abc/1
  A/1 -> Product2/1, Product1/1, Product/1
  Product/1 -> Mux/1
  Product1/1 -> Mux/2
  Product2/1 -> Mux/3
  Trigonometric Function2/1 -> Product2/2
  Trigonometric Function1/1 -> Product1/2
  Trigonometric Function/1 -> Product/2
  Sum1/1 -> Trigonometric Function2/1
  Sum/1 -> Trigonometric Function1/1
  Sum2/1 -> Sum/1, Sum1/1, Trigonometric Function/1
  Integrator/1 -> Sum2/1
  Constant2/1 -> Sum3/2
  Sum3/1 -> Integrator/1
  Step/1 -> Rate Limiter/1

== system DetailedModel/ powerline/ 0 km ==
  note: L2
  A1 : PMIOPort  Side=Left
  B1 : PMIOPort  Port=2  Side=Left
  C1 : PMIOPort  Port=3  Side=Left
  A2 : PMIOPort  Port=4  Side=Right
  B2 : PMIOPort  Port=5  Side=Right
  C2 : PMIOPort  Port=6  Side=Right
  connections:
  A1/RConn1 -- A2/RConn1
  B1/RConn1 -- B2/RConn1
  C1/RConn1 -- C2/RConn1

== system DetailedModel/ powerline/ 0.5 km ==
  note: L2
  note: L1
  Ground : spsGroundLib/Ground  LConnTagsString=a
  Three-Phase Series RLC Branch1 : spsThreePhaseSeriesRLCBranchLib/Three-Phase Series RLC Branch  LConnTagsString=A|B|C  RConnTagsString=A|B|C  BranchType=RL  Resistance=R  Inductance=L  Capacitance=1e-6  Measurements=None
  Three-Phase Series RLC Branch2 : spsThreePhaseSeriesRLCBranchLib/Three-Phase Series RLC Branch  LConnTagsString=A|B|C  RConnTagsString=A|B|C  BranchType=C  Resistance=inv.RC  Inductance=13e-6  Capacitance=C  Measurements=None
  Three-Phase Series RLC Branch3 : spsThreePhaseSeriesRLCBranchLib/Three-Phase Series RLC Branch  LConnTagsString=A|B|C  RConnTagsString=A|B|C  BranchType=C  Resistance=inv.RC  Inductance=13e-6  Capacitance=C  Measurements=None
  A1 : PMIOPort  Side=Left
  B1 : PMIOPort  Port=2  Side=Left
  C1 : PMIOPort  Port=3  Side=Left
  A2 : PMIOPort  Port=4  Side=Right
  B2 : PMIOPort  Port=5  Side=Right
  C2 : PMIOPort  Port=6  Side=Right
  connections:
  Three-Phase Series RLC Branch2/LConn3 -- Three-Phase Series RLC Branch1/RConn1 -- A2/RConn1
  A1/RConn1 -- Three-Phase Series RLC Branch1/LConn1 -- Three-Phase Series RLC Branch3/LConn3
  Three-Phase Series RLC Branch2/LConn2 -- Three-Phase Series RLC Branch1/RConn2 -- B2/RConn1
  B1/RConn1 -- Three-Phase Series RLC Branch1/LConn2 -- Three-Phase Series RLC Branch3/LConn2
  Three-Phase Series RLC Branch1/RConn3 -- Three-Phase Series RLC Branch2/LConn1 -- C2/RConn1
  C1/RConn1 -- Three-Phase Series RLC Branch1/LConn3 -- Three-Phase Series RLC Branch3/LConn1
  Three-Phase Series RLC Branch2/RConn2 -- Three-Phase Series RLC Branch2/RConn3 -- Three-Phase Series RLC Branch2/RConn1 -- Ground/LConn1 -- Three-Phase Series RLC Branch3/RConn3 -- Three-Phase Series RLC Branch3/RConn2 -- Three-Phase Series RLC Branch3/RConn1
